simulink model "Drehteller"  (R2021b)
settings: Solver=ode3  StartTime=0.0  StopTime=10.0  FixedStep=0.01  RelTol=1e-3
values from neighbouring files (symbols this model uses):
  A = 5    [Parametriesierung.m]
  I = 0.5    [Parametriesierung.m]
  igetr = 1080    [Parametriesierung.m]
  K = 8    [Parametriesierung.m]
  MRK = 1    [Parametriesierung.m]
  PHI = 0.001    [Parametriesierung.m]
  Ra = 40    [Parametriesierung.m]
  U = 24    [Parametriesierung.m]
settings Model: Creator=mwjae  LastModifiedBy=mwjae

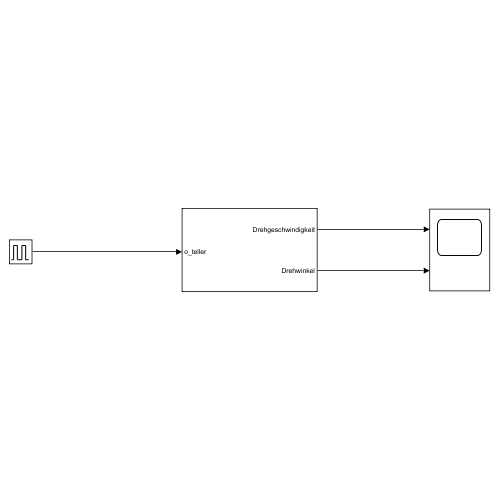
[thumbnail: Simulink's stored preview of the top-level diagram]
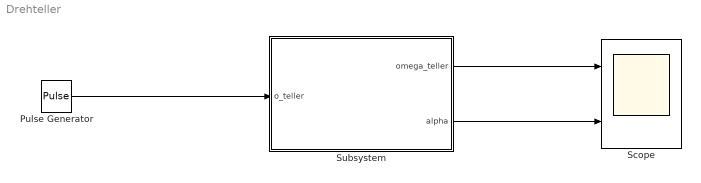
== system Drehteller ==
  Pulse Generator : DiscretePulseGenerator  PulseType=Time based  PulseWidth=50
  Scope : Scope  NumInputPorts=2
  Subsystem : Subsystem
  wires:
  Pulse Generator/1 -> Subsystem/1(o_teller)
  Subsystem/1(omega_teller) -> Scope/1
  Subsystem/2(alpha) -> Scope/2

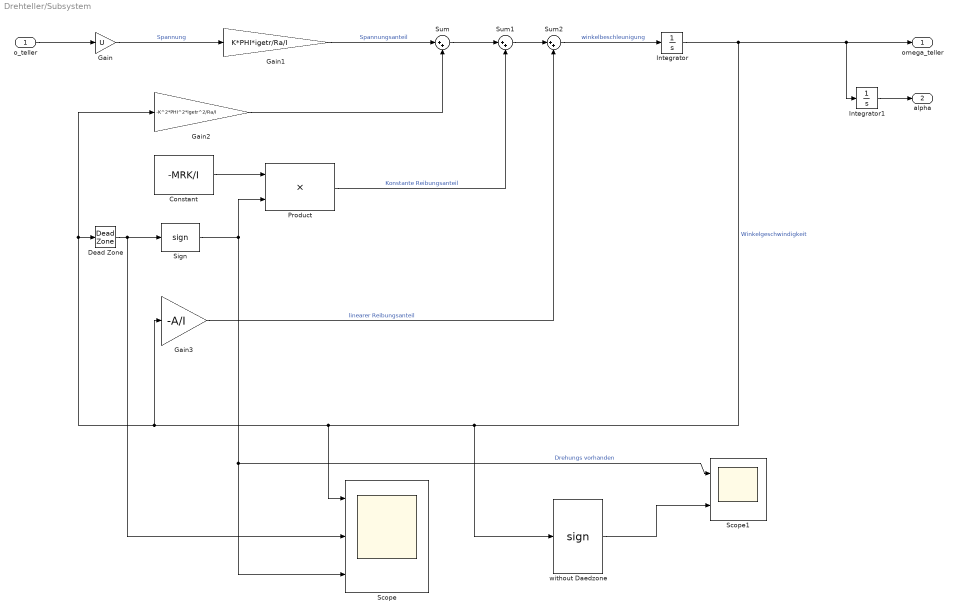
== system Drehteller/Subsystem ==
  o_teller : Inport
  Constant : Constant  Value=-MRK/I
  Dead Zone : DeadZone  SaturateOnIntegerOverflow=on
  Gain : Gain  Gain=U
  Gain1 : Gain  Gain=K*PHI*igetr/Ra/I
  Gain2 : Gain  Gain=-K^2*PHI^2*igetr^2/Ra/I
  Gain3 : Gain  Gain=-A/I
  Integrator : Integrator
  Integrator1 : Integrator
  Product : Product
  Scope : Scope  NumInputPorts=3
  Scope1 : Scope  NumInputPorts=2
  Sign : Signum
  Sum : Sum  Inputs=|++
  Sum1 : Sum  Inputs=|++
  Sum2 : Sum  Inputs=|++
  without Daedzone : Signum
  omega_teller : Outport
  alpha : Outport  Port=2
  wires:
  o_teller/1 -> Gain/1
  Gain/1 -> Gain1/1  "Spannung"
  Constant/1 -> Product/1
  Dead Zone/1 -> Scope/2, Sign/1
  Gain3/1 -> Sum2/2  "linearer Reibungsanteil"
  Product/1 -> Sum1/2  "Konstante Reibungsanteil"
  Gain1/1 -> Sum/1  "Spannungsanteil"
  Gain2/1 -> Sum/2
  Sum/1 -> Sum1/1
  Sum1/1 -> Sum2/1
  Sum2/1 -> Integrator/1  "winkelbeschleunigung"
  Integrator/1 -> without Daedzone/1, Scope/1, Gain3/1, Gain2/1, Dead Zone/1, Integrator1/1, omega_teller/1  "Winkelgeschwindigkeit"
  Integrator1/1 -> alpha/1
  without Daedzone/1 -> Scope1/2
  Sign/1 -> Scope/3, Scope1/1, Product/2  "Drehungs vorhanden"
